simulink model "two_dof_example"  (R2025a)
settings: Solver=daessc  StartTime=0.0  StopTime=5  MaxStep=1e-2  RelTol=1e-3
libraries: fl_lib x10, nesl_utility x8, sdl_lib x2
settings Model: Creator=mtpanny  LastModifiedBy=mtpanny

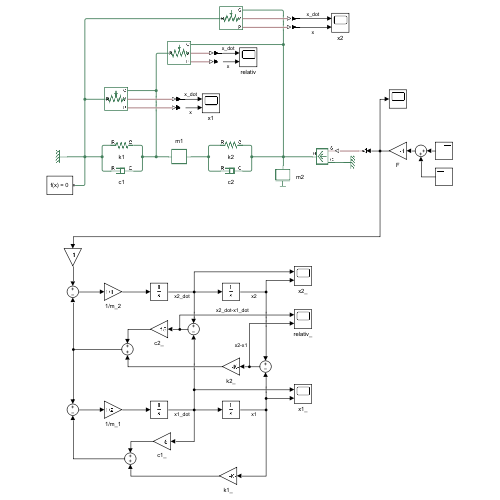
[thumbnail: Simulink's stored preview of the top-level diagram]
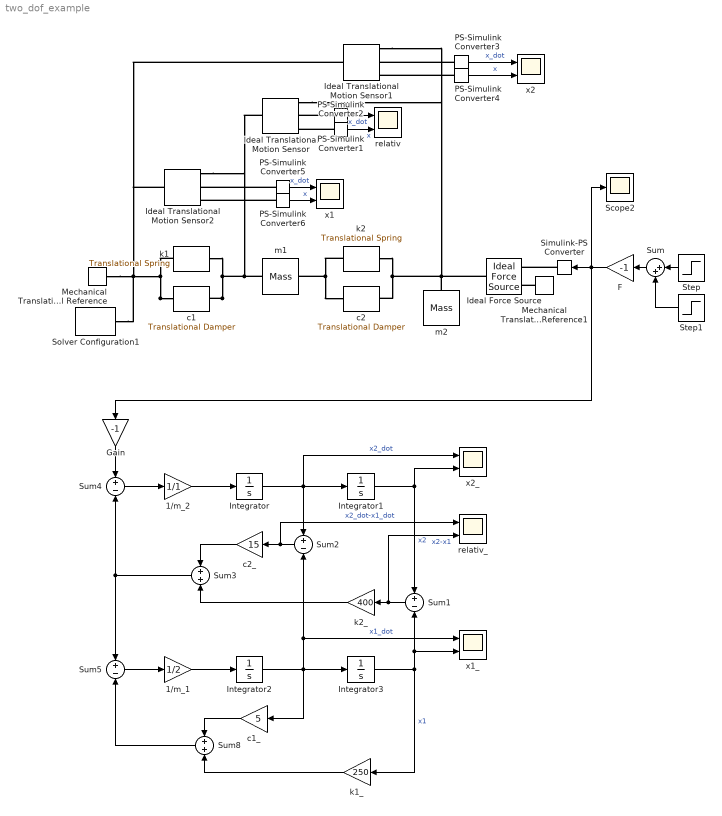
== system two_dof_example ==
  1/m_1 : Gain  Gain=1/2
  1/m_2 : Gain  Gain=1/1
  F : Gain  Gain=-1
  Gain : Gain  Gain=-1
  Ideal Force Source : fl_lib/Mechanical/Mechanical Sources/Ideal Force Source
  Ideal Translational Motion Sensor : fl_lib/Mechanical/Mechanical Sensors/Ideal Translational Motion Sensor  reference=foundation.enum.MeasurementReference.difference  acceleration_port=false  velocity_port=true  position_port=true  offset=0 m
  Ideal Translational Motion Sensor1 : fl_lib/Mechanical/Mechanical Sensors/Ideal Translational Motion Sensor  reference=foundation.enum.MeasurementReference.difference  acceleration_port=false  velocity_port=true  position_port=true  offset=0 m
  Ideal Translational Motion Sensor2 : fl_lib/Mechanical/Mechanical Sensors/Ideal Translational Motion Sensor  reference=foundation.enum.MeasurementReference.difference  acceleration_port=false  velocity_port=true  position_port=true  offset=0 m
  Integrator{,1..3} (4 alike) : Integrator
  Mechanical Translational Reference : fl_lib/Mechanical/Translational Elements/Mechanical Translational Reference
  Mechanical Translational Reference1 : fl_lib/Mechanical/Translational Elements/Mechanical Translational Reference
  PS-Simulink Converter{1..6} (6 alike) : nesl_utility/PS-Simulink Converter  PhysicalDomain=network_engine_domain  SubClassName=ps_output  LeftPortType=input  RightPortType=output  PseudoPeriodic=off  Frequencies=[]  VectorFormat=inherit  Unit=inherit  AffineConversion=off
  Scope2 : Scope
      settings: ActiveDisplayYMinimum=-1  ActiveDisplayYMaximum=1  DataLoggingVariableName=ScopeData2
  Simulink-PS Converter : nesl_utility/Simulink-PS Converter  PhysicalDomain=network_engine_domain  SubClassName=ps_input  LeftPortType=input  RightPortType=output  PseudoPeriodic=off  Frequencies=[]  NoiseDistribution=none  NoiseParameters=[]  Unit=1  AffineConversion=off  FilteringAndDerivatives=provide  SimscapeFilterOrder=1  InputFilterTimeConstant=0.001  UdotUserProvided=0
  Solver Configuration1 : nesl_utility/Solver Configuration  PhysicalDomain=network_engine_domain  SubClassName=solver  LeftPortType=input  RightPortType=generic  Tones=[]  Harmonics=[]  SimulateNoise=off  Profile=off  UseLocalSampling=off  EnableSwitchedLinearOptims=on  FrequencyDomain=off  UseCCode=off  RelTol=0.001  AbsTol=0.001  MinStep=1e-09  ToWorkspace=off  RevertToSquareIcSolve=off  NumHomotopyIterations=100  PhasorMode=off  PhasorModeNumHarmonics=1  ConsistencySolver=NEWTON_XTOL_AFTER_FTOL  IndexReductionMethod=DerivativeReplacement  DoDC=off  ResidualTolerance=1e-09  ConsistencyTolSource=GLOBAL  ConsistencyAbsTol=0.001  ConsistencyRelTol=0.001  ConsistencyTolFactor=0.001  UseLocalSolver=off  LocalSolverChoice=NE_BACKWARD_EULER_ADVANCER  ResolveIndetEquations=on  FunctionEvalNumThread=1  LocalSolverSampleTime=0.001  DoFixedCost=off  MaxNonlinIter=3  MaxModeIter=2  ComputeImpulses=off  ImpulseIterations=2  LinearAlgebra=auto  LinearAlgebraNumThread=0  EquationFormulation=NE_TIME_EF  DelaysMemoryBudget=1024  AutomaticFiltering=on  FilteringTimeConstant=0.001  PartitionStorageMethod=AS_NEEDED  PartitionMemoryBudget=1024  PartitionMethod=ROBUST  MultibodyUseLocalSolver=off  MultibodyLocalSolverChoice=ODE1  MultibodyLocalSolverSampleTime=0.001
  Step : Step  Time=5/4  SampleTime=0
  Step1 : Step  Time=5/4*3  After=-1  SampleTime=0
  Sum : Sum  Inputs=|++
  Sum{1..2,4..5} (4 alike) : Sum  Inputs=+|-
  Sum3 : Sum  Inputs=+|+
  Sum8 : Sum  Inputs=+|+
  c1 : sdl_lib/Couplings & Drives/Springs & Dampers/Translational Damper  D=5 N*s/m  thermal_port=simscape.enum.thermaleffects.omit  thermal_mass=50 kJ/K  temperature_specify=off  temperature_priority=High  temperature=300 K  temperature_nominal_specify=off  temperature_nominal_value=1  temperature_nominal_unit=K
  c1_ : Gain  Gain=5
  c2 : sdl_lib/Couplings & Drives/Springs & Dampers/Translational Damper  D=15 N*s/m  thermal_port=simscape.enum.thermaleffects.omit  thermal_mass=50 kJ/K  temperature_specify=off  temperature_priority=High  temperature=300 K  temperature_nominal_specify=off  temperature_nominal_value=1  temperature_nominal_unit=K
  c2_ : Gain  Gain=15
  k1 : fl_lib/Mechanical/Translational Elements/Translational Spring  spr_rate=250 N/m  v_specify=off  v_priority=None  v=0 m/s  v_nominal_specify=off  v_nominal_value=1  v_nominal_unit=m/s  f_specify=off  f_priority=None  f=0 N  f_nominal_specify=off  f_nominal_value=1  f_nominal_unit=N  x_specify=off  x_priority=High  x=1 m  x_nominal_specify=off  x_nominal_value=1  x_nominal_unit=m
  k1_ : Gain  Gain=250
  k2 : fl_lib/Mechanical/Translational Elements/Translational Spring  spr_rate=400 N/m  v_specify=off  v_priority=None  v=0 m/s  v_nominal_specify=off  v_nominal_value=1  v_nominal_unit=m/s  f_specify=off  f_priority=None  f=0 N  f_nominal_specify=off  f_nominal_value=1  f_nominal_unit=N  x_specify=off  x_priority=High  x=1 m  x_nominal_specify=off  x_nominal_value=1  x_nominal_unit=m
  k2_ : Gain  Gain=400
  m1 : fl_lib/Mechanical/Translational Elements/Mass  mass=2 kg  num_ports=foundation.enum.numPorts2.two  v_specify=off  v_priority=High  v=0 m/s  v_nominal_specify=off  v_nominal_value=1  v_nominal_unit=m/s  f_specify=off  f_priority=None  f=0 N  f_nominal_specify=off  f_nominal_value=1  f_nominal_unit=N
      settings: InternalSimscapePortConfiguration="{\"Bottom\":[],\"Left\":[{\"id\":\"M\",\"label\":\"\",\"type\":\"foundation.mechanical.translational.translational\"}],\"Right\":[{\"id\":\"N\",\"label\":\"\",\"type\":\"foundation.mechanical.translational.translational\"}],\"Top\":[]}"
  m2 : fl_lib/Mechanical/Translational Elements/Mass  mass=1 kg  num_ports=foundation.enum.numPorts2.one  v_specify=off  v_priority=High  v=0 m/s  v_nominal_specify=off  v_nominal_value=1  v_nominal_unit=m/s  f_specify=off  f_priority=None  f=0 N  f_nominal_specify=off  f_nominal_value=1  f_nominal_unit=N
  relativ : Scope  NumInputPorts=2
      settings: ActiveDisplayYMinimum=-0.027701519177981568  ActiveDisplayYMaximum=0.027468994487329531
  relativ_ : Scope  NumInputPorts=2
      settings: ActiveDisplayYMinimum=-0.029805664159759632  ActiveDisplayYMaximum=0.029642805711890406  DataLoggingVariableName=ScopeData6
  x1 : Scope  NumInputPorts=2
      settings: ActiveDisplayYMinimum=-0.0491066409804823  ActiveDisplayYMaximum=0.04485753753710682  DataLoggingVariableName=ScopeData3
  x1_ : Scope  NumInputPorts=2
      settings: ActiveDisplayYMinimum=-0.050040764049698871  ActiveDisplayYMaximum=0.045704032039770977  DataLoggingVariableName=ScopeData5
  x2 : Scope  NumInputPorts=2
      settings: ActiveDisplayYMinimum=-0.056195090318118424  ActiveDisplayYMaximum=0.050992557355003271
  x2_ : Scope  NumInputPorts=2
      settings: ActiveDisplayYMinimum=-0.050971349151717728  ActiveDisplayYMaximum=0.055995922104007584  DataLoggingVariableName=ScopeData4
  wires:
  PS-Simulink Converter1/1 -> relativ/1  "x_dot"
  PS-Simulink Converter2/1 -> relativ/2  "x"
  Step/1 -> Sum/1
  Step1/1 -> Sum/2
  Sum/1 -> F/1
  F/1 -> Scope2/1, Gain/1, Simulink-PS Converter/1
  PS-Simulink Converter4/1 -> x2/2  "x"
  PS-Simulink Converter3/1 -> x2/1  "x_dot"
  PS-Simulink Converter6/1 -> x1/2  "x"
  PS-Simulink Converter5/1 -> x1/1  "x_dot"
  Integrator/1 -> x2_/1, Integrator1/1, Sum2/1  "x2_dot"
  Integrator1/1 -> x2_/2, Sum1/1  "x2"
  Sum1/1 -> relativ_/2, k2_/1  "x2-x1"
  Sum2/1 -> relativ_/1, c2_/1  "x2_dot-x1_dot"
  c2_/1 -> Sum3/1
  k2_/1 -> Sum3/2
  Sum4/1 -> 1/m_2/1
  Sum3/1 -> Sum4/2, Sum5/1
  Sum5/1 -> 1/m_1/1
  k1_/1 -> Sum8/2
  c1_/1 -> Sum8/1
  Integrator2/1 -> Sum2/2, x1_/1, Integrator3/1, c1_/1  "x1_dot"
  Integrator3/1 -> x1_/2, Sum1/2, k1_/1  "x1"
  1/m_1/1 -> Integrator2/1
  1/m_2/1 -> Integrator/1
  Sum8/1 -> Sum5/2
  Gain/1 -> Sum4/1
  connections:
  c1/RConn1 -- Ideal Translational Motion Sensor2/RConn1 -- Ideal Translational Motion Sensor/LConn1 -- m1/LConn1 -- k1/RConn1
  c1/LConn1 -- k1/LConn1 -- Ideal Translational Motion Sensor1/LConn1 -- Ideal Translational Motion Sensor2/LConn1 -- Solver Configuration1/RConn1 -- Mechanical Translational Reference/LConn1
  PS-Simulink Converter1/LConn1 -- Ideal Translational Motion Sensor/RConn2
  PS-Simulink Converter2/LConn1 -- Ideal Translational Motion Sensor/RConn3
  k2/RConn1 -- Ideal Translational Motion Sensor/RConn1 -- Ideal Translational Motion Sensor1/RConn1 -- m2/LConn1 -- Ideal Force Source/LConn1 -- c2/RConn1
  k2/LConn1 -- m1/RConn1 -- c2/LConn1
  Mechanical Translational Reference1/LConn1 -- Ideal Force Source/RConn2
  Simulink-PS Converter/RConn1 -- Ideal Force Source/RConn1
  PS-Simulink Converter4/LConn1 -- Ideal Translational Motion Sensor1/RConn3
  PS-Simulink Converter3/LConn1 -- Ideal Translational Motion Sensor1/RConn2
  PS-Simulink Converter6/LConn1 -- Ideal Translational Motion Sensor2/RConn3
  PS-Simulink Converter5/LConn1 -- Ideal Translational Motion Sensor2/RConn2
